simulink library "Star_delta_StarterV2"  (R2024a)
settings: Solver=VariableStepAuto  StartTime=0.0  StopTime=10.0  RelTol=1e-3
libraries: spsThreePhaseBreakerLib x3, simulink_extras x1
settings Model: Creator=gshma  LastModifiedBy=gshma

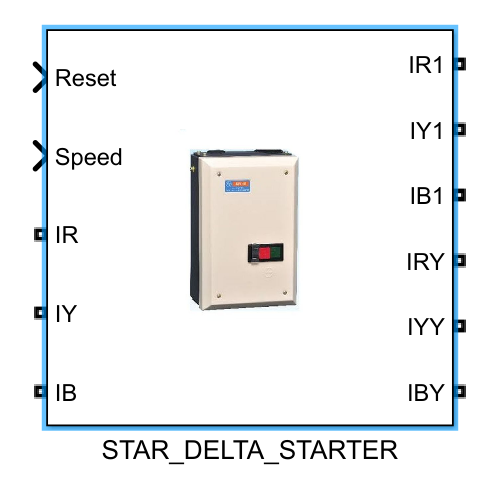
[thumbnail: Simulink's stored preview of the top-level diagram]
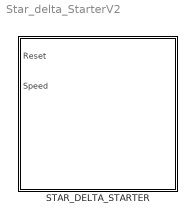
== system Star_delta_StarterV2 ==
  STAR_DELTA_STARTER : Subsystem
      mask Display: image('star_delt.jpg', [0,0,0,0,50,50]);

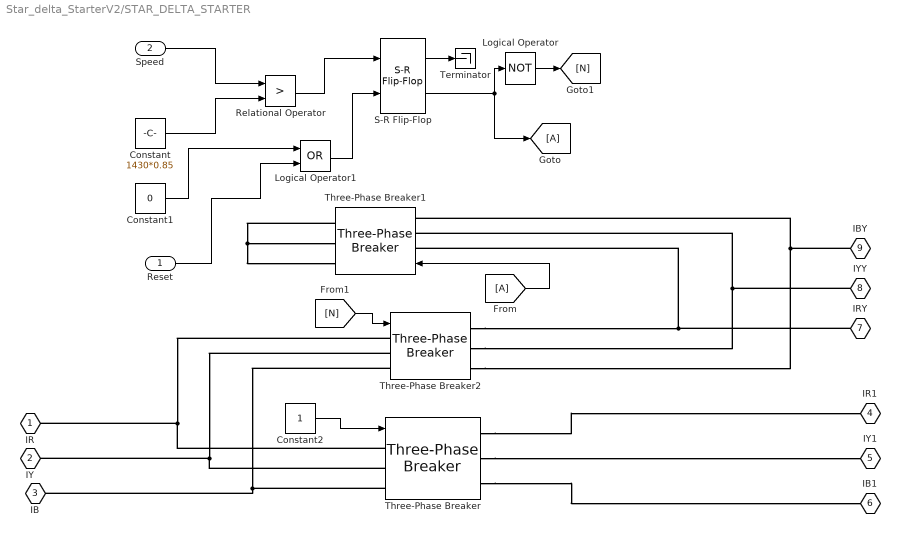
== system Star_delta_StarterV2/STAR_DELTA_STARTER ==
  Reset : Inport
  Speed : Inport  Port=2
  Constant : Constant  Value=1430*0.85
  Constant1 : Constant  Value=0  OutDataTypeStr=boolean
  Constant2 : Constant  OutDataTypeStr=boolean
  From : From
  Goto : Goto
  Logical Operator : Logic  Operator=NOT  AllPortsSameDT=off  OutDataTypeStr=boolean
  Logical Operator1 : Logic  Operator=OR  AllPortsSameDT=off  OutDataTypeStr=boolean
  Relational Operator : RelationalOperator  Operator=>  OutDataTypeStr=boolean  RndMeth=Simplest  InputSameDT=off
  S-R Flip-Flop : simulink_extras/Flip Flops/S-R Flip-Flop  initial_condition=0
  Terminator : Terminator
  Three-Phase Breaker : spsThreePhaseBreakerLib/Three-Phase Breaker  InitialState=closed  SwitchA=on  SwitchB=on  SwitchC=on  SwitchTimes="[1/60  5/60]"  External=on  BreakerResistance=0.01  SnubberResistance=1e6  SnubberCapacitance=inf  Measurements=None
  Three-Phase Breaker1 : spsThreePhaseBreakerLib/Three-Phase Breaker  InitialState=closed  SwitchA=on  SwitchB=on  SwitchC=on  SwitchTimes="[1/60  5/60]"  External=on  BreakerResistance=0.01  SnubberResistance=1e6  SnubberCapacitance=inf  Measurements=None
  Three-Phase Breaker2 : spsThreePhaseBreakerLib/Three-Phase Breaker  InitialState=open  SwitchA=on  SwitchB=on  SwitchC=on  SwitchTimes="[1/60  5/60]"  External=on  BreakerResistance=0.01  SnubberResistance=1e6  SnubberCapacitance=inf  Measurements=None
  IR : PMIOPort  Tag=simrfV2util1/Connection Port  Side=Left
  IY : PMIOPort  Tag=simrfV2util1/Connection Port  Port=2  Side=Left
  IB : PMIOPort  Tag=simrfV2util1/Connection Port  Port=3  Side=Left
  IR1 : PMIOPort  Tag=simrfV2util1/Connection Port  Port=4  Side=Right
  IY1 : PMIOPort  Tag=simrfV2util1/Connection Port  Port=5  Side=Right
  IB1 : PMIOPort  Tag=simrfV2util1/Connection Port  Port=6  Side=Right
  IRY : PMIOPort  Tag=simrfV2util1/Connection Port  Port=7  Side=Right
  IYY : PMIOPort  Tag=simrfV2util1/Connection Port  Port=8  Side=Right
  IBY : PMIOPort  Tag=simrfV2util1/Connection Port  Port=9  Side=Right
  wires:
  Relational Operator/1 -> S-R Flip-Flop/1
  S-R Flip-Flop/1 -> Terminator/1
  Logical Operator1/1 -> S-R Flip-Flop/2
  S-R Flip-Flop/2 -> Goto/1, Logical Operator/1
  Logical Operator/1 -> [N]
  From/1 -> Three-Phase Breaker1/1
  [N] -> Three-Phase Breaker2/1
  Constant2/1 -> Three-Phase Breaker/1
  Reset/1 -> Logical Operator1/2
  Speed/1 -> Relational Operator/1
  Constant/1 -> Relational Operator/2
  Constant1/1 -> Logical Operator1/1
  connections:
  IR/RConn1 -- Three-Phase Breaker2/LConn1 -- Three-Phase Breaker/LConn1
  Three-Phase Breaker/LConn2 -- IY/RConn1 -- Three-Phase Breaker2/LConn2
  Three-Phase Breaker/LConn3 -- IB/RConn1 -- Three-Phase Breaker2/LConn3
  Three-Phase Breaker/RConn1 -- IR1/RConn1
  Three-Phase Breaker/RConn2 -- IY1/RConn1
  Three-Phase Breaker/RConn3 -- IB1/RConn1
  Three-Phase Breaker1/RConn3 -- Three-Phase Breaker1/RConn1 -- Three-Phase Breaker1/RConn2
  IBY/RConn1 -- Three-Phase Breaker2/RConn3 -- Three-Phase Breaker1/LConn3
  IYY/RConn1 -- Three-Phase Breaker2/RConn2 -- Three-Phase Breaker1/LConn2
  IRY/RConn1 -- Three-Phase Breaker2/RConn1 -- Three-Phase Breaker1/LConn1
